simulink model "Experimento3"  (R2023a)
settings: Solver=ode4  StartTime=0.0  StopTime=10.0  FixedStep=0.01  RelTol=1e-3
undefined symbols (not defined in the file): G5
settings Model: Creator=carlo  LastModifiedBy=carlo

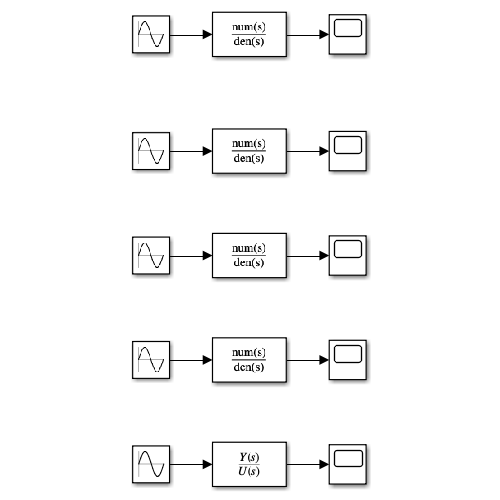
[thumbnail: Simulink's stored preview of the top-level diagram]
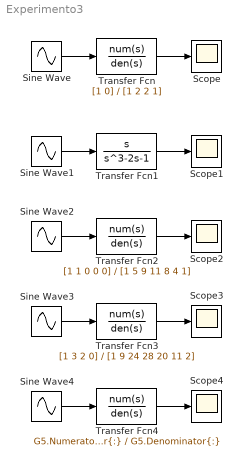
== system Experimento3 ==
  Scope{,1..4} (5 alike) : Scope
  Sine Wave{,1..4} (5 alike) : Sin  Frequency=2  SampleTime=0
  Transfer Fcn : TransferFcn  Numerator=[1 0]  Denominator=[1 2 2 1]
  Transfer Fcn1 : TransferFcn  Numerator=[1 0]  Denominator=[1 0 -2 -1]
  Transfer Fcn2 : TransferFcn  Numerator=[1 1 0 0 0]  Denominator=[1 5 9 11 8 4 1]
  Transfer Fcn3 : TransferFcn  Numerator=[1 3 2 0]  Denominator=[1 9 24 28 20 11 2]
  Transfer Fcn4 : TransferFcn  Numerator=G5.Numerator{:}  Denominator=G5.Denominator{:}
  wires:
  Sine Wave/1 -> Transfer Fcn/1
  Transfer Fcn/1 -> Scope/1
  Transfer Fcn1/1 -> Scope1/1
  Sine Wave1/1 -> Transfer Fcn1/1
  Sine Wave2/1 -> Transfer Fcn2/1
  Transfer Fcn2/1 -> Scope2/1
  Transfer Fcn3/1 -> Scope3/1
  Sine Wave3/1 -> Transfer Fcn3/1
  Sine Wave4/1 -> Transfer Fcn4/1
  Transfer Fcn4/1 -> Scope4/1
